simulink model "modelo_real"  (R2018b)
settings: Solver=ode4  StartTime=0.0  StopTime=t_f  FixedStep=fst  RelTol=1e-3  EnableMultiTasking=on
values from neighbouring files (symbols this model uses):
  b = 0.1210    (= 0.121)    [Script_principal.m]
  c_d = r_d/(2*b)    (= 0.120661157025)    [Script_principal.m]
  c_e = r_e/(2*b)    (= 0.121074380165)    [Script_principal.m]
  delayD = 0.1/fst    (= 100)    [Script_principal.m]
  delayE = 0.1/fst    (= 100)    [Script_principal.m]
  fD_v = var_fD*0.0069    (= 0.0069)    [Script_principal.m]
  fE_v = var_fE*0.0053    (= 0.0053)    [Script_principal.m]
  filter_order = 2    [Script_principal.m]
  freq_pos = 200    [Script_principal.m]
  freq_vel = 200    [Script_principal.m]
  I_v = var_I*0.0903    (= 0.0903)    [Script_principal.m]
  Ir_v = var_Ir*0.00094    (= 0.00094)    [Script_principal.m]
  k0 = 25    [Script_principal.m]
  k1 = 25    [Script_principal.m]
  k_enc = 2*pi/fpr    (= 0.157079632679)    [Script_principal.m]
  KaD_v = var_KaD*0.4713    (= 0.4713)    [Script_principal.m]
  KaE_v = var_KaE*0.5046    (= 0.5046)    [Script_principal.m]
  KtD_v = var_KtD*KaD    (= 0.4713)    [Script_principal.m]
  KtE_v = var_KtE*KaE    (= 0.5046)    [Script_principal.m]
  L = 0.10    (= 0.1)    [Script_principal.m]
  m_v = var_m*1.932    (= 1.932)    [Script_principal.m]
  r_d = 0.0292    [Script_principal.m]
  r_e = 0.0293    [Script_principal.m]
  RaD_v = var_RaD*8.4507    (= 8.4507)    [Script_principal.m]
  RaE_v = var_RaE*7.7177    (= 7.7177)    [Script_principal.m]
  svzD = 0    [Script_principal.m]
  svzE = 0    [Script_principal.m]
  T = 4    [Script_principal.m]
  VaD_max = 14    [Script_principal.m]
  VaD_min = 2    [Script_principal.m]
  VaE_max = 14    [Script_principal.m]
  VaE_min = 2    [Script_principal.m]
  x0_1 = 0    [Script_principal.m]
  x0_2 = -L    (= -0.1)    [Script_principal.m]
  x0_3 = (pi/2)/c_d    (= 13.0182435303)    [Script_principal.m]
  x0_4 = 0    [Script_principal.m]
  x0_5 = 0    [Script_principal.m]
  x0_6 = 0    [Script_principal.m]
undefined symbols (not defined in the file or in its folder): a, dur_c, t_f, t_i, t_i_1, t_i_2, t_i_3, t_i_c, time_c, v, w, wx, wy
libraries: simulink x39, embdlinuxlib x7, dspmtrx3 x6, cstblocks x4, raspberrypilib x1
(part 1 of 2)
settings Model: SimulationMode=external  ExtModeTrigDuration=2  Creator=nenem  LastModifiedBy=nenem
settings SolverCC: PositivePriorityOrder=on
settings OptimizationCC: EnhancedBackFolding=on  PassReuseOutputArgsAs=Individual arguments  MaxStackSize=64  OptimizeBlockOrder=speed  DifferentSizesBufferReuse=on  OptimizationCustomize=off
settings DebuggingCC: ParameterTunabilityLossMsg=error
settings HardwareCC: ProdBitPerPointer=32  ProdBitPerSizeT=32  ProdBitPerPtrDiffT=32  ProdLargestAtomicInteger=Long  ProdLargestAtomicFloat=Double  ProdWordSize=32  ProdHWDeviceType=ARM Compatible->ARM Cortex
settings SFSimCC: MATLABDynamicMemAlloc=off
settings RTWCC: SystemTargetFile=ert.tlc  HardwareBoard=Raspberry Pi  TLCOptions="-aInlineSetEventsForThisBaseRateFcn=TLC_FALSE -aSuppressMultiTaskScheduler=TLC_FALSE  -aRateBasedStepFcn=0"  TemplateMakefile=ert_default_tmf  GenerateReport=on  Toolchain=GNU GCC Raspberry Pi  BuildConfiguration=Faster Runs  IncludeHyperlinkInReport=on  LaunchReport=on  GenerateTraceInfo=on  GenerateTraceReport=on  GenerateTraceReportSl=on  GenerateTraceReportSf=on  GenerateTraceReportEml=on
settings CodeAppCC: ForceParamTrailComments=on  IgnoreCustomStorageClasses=off  OperatorAnnotations=on  SimulinkDataObjDesc=on  SFDataObjDesc=on  InsertBlockDesc=on
settings ERTTargetCC: SupportContinuousTime=on  SupportVariableSizeSignals=on

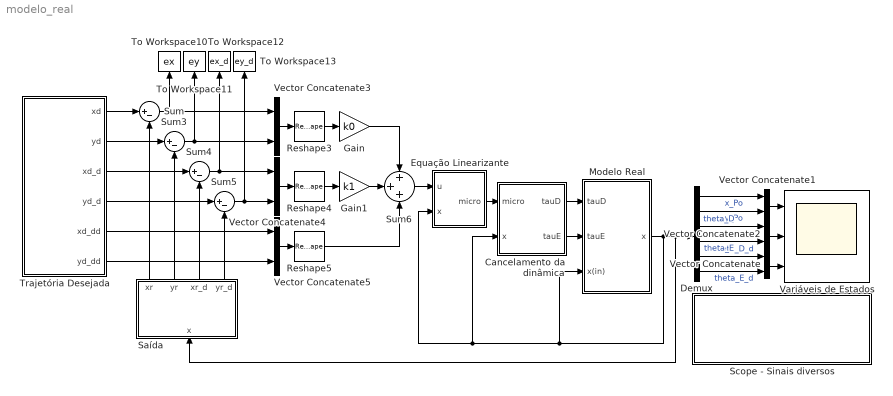
== system modelo_real ==
  Cancelamento da dinâmica : Subsystem
  Demux : Demux  Outputs=6
  Equação Linearizante : Subsystem
  Gain : Gain  Gain=k0
  Gain1 : Gain  Gain=k1
  Modelo Real : Subsystem
  Reshape3 : Reshape  OutputDimensionality=Customize  OutputDimensions=[2,1]
  Reshape4 : Reshape  OutputDimensionality=Customize  OutputDimensions=[2,1]
  Reshape5 : Reshape  OutputDimensionality=Customize  OutputDimensions=[2,1]
  Saída : Subsystem
  Scope - Sinais diversos : Subsystem
  Sum{,3..5} (4 alike) : Sum  Inputs=|+-
  Sum6 : Sum  Inputs=+++
  To Workspace10 : ToWorkspace  VariableName=ex  SaveFormat=Structure With Time  SampleTime=-1
      settings: Save2DSignal=2-D array (concatenate along first dimension)
  To Workspace11 : ToWorkspace  VariableName=ey  SaveFormat=Structure With Time  SampleTime=-1
      settings: Save2DSignal=2-D array (concatenate along first dimension)
  To Workspace12 : ToWorkspace  VariableName=ex_d  SaveFormat=Structure With Time  SampleTime=-1
      settings: Save2DSignal=2-D array (concatenate along first dimension)
  To Workspace13 : ToWorkspace  VariableName=ey_d  SaveFormat=Structure With Time  SampleTime=-1
      settings: Save2DSignal=2-D array (concatenate along first dimension)
  Trajetória Desejada : Subsystem
  Variáveis de Estados : Scope  NumInputPorts=3
  Vector Concatenate{,1..5} (6 alike) : Concatenate
  wires:
  Trajetória Desejada/4(yd_d) -> Sum5/1
  Vector Concatenate5/1 -> Reshape5/1
  Vector Concatenate3/1 -> Reshape3/1
  Vector Concatenate4/1 -> Reshape4/1
  Reshape3/1 -> Gain/1
  Gain/1 -> Sum6/1
  Gain1/1 -> Sum6/2
  Trajetória Desejada/3(xd_d) -> Sum4/1
  Trajetória Desejada/6(yd_dd) -> Vector Concatenate5/2
  Trajetória Desejada/5(xd_dd) -> Vector Concatenate5/1
  Reshape5/1 -> Sum6/3
  Reshape4/1 -> Gain1/1
  Equação Linearizante/1(micro) -> Cancelamento da dinâmica/1(micro)
  Sum6/1 -> Equação Linearizante/1(u)
  Trajetória Desejada/1(xd) -> Sum/1
  Trajetória Desejada/2(yd) -> Sum3/1
  Modelo Real/1(x) -> Saída/1(x), Demux/1, Modelo Real/3(x(in)), Cancelamento da dinâmica/2(x), Equação Linearizante/2(x)
  Vector Concatenate2/1 -> Variáveis de Estados/2
  Vector Concatenate1/1 -> Variáveis de Estados/1
  Vector Concatenate/1 -> Variáveis de Estados/3
  Demux/1 -> Vector Concatenate1/1  "x_Po"
  Demux/2 -> Vector Concatenate1/2  "y_Po"
  Demux/5 -> Vector Concatenate/1  "theta_D_d"
  Demux/6 -> Vector Concatenate/2  "theta_E_d"
  Demux/4 -> Vector Concatenate2/2  "theta_E"
  Demux/3 -> Vector Concatenate2/1  "theta_D"
  Cancelamento da dinâmica/1(tauD) -> Modelo Real/1(tauD)
  Cancelamento da dinâmica/2(tauE) -> Modelo Real/2(tauE)
  Saída/1(xr) -> Sum/2
  Saída/2(yr) -> Sum3/2
  Saída/3(xr_d) -> Sum4/2
  Saída/4(yr_d) -> Sum5/2
  Sum3/1 -> Vector Concatenate3/2, To Workspace11/1
  Sum/1 -> Vector Concatenate3/1, To Workspace10/1
  Sum4/1 -> To Workspace12/1, Vector Concatenate4/1
  Sum5/1 -> Vector Concatenate4/2, To Workspace13/1

== system modelo_real/Cancelamento da dinâmica ==
  micro : Inport
  x : Inport  Port=2
  Constant1 : Constant  Value=[b r_d r_e c_d c_e Ir_v m_v I_v]
  Reshape7 : Reshape  OutputDimensionality=Customize  OutputDimensions=[1,8]
  To Workspace18 : ToWorkspace  VariableName=tauD  SaveFormat=Structure With Time  SampleTime=-1
      settings: Save2DSignal=2-D array (concatenate along first dimension)
  To Workspace19 : ToWorkspace  VariableName=tauE  SaveFormat=Structure With Time  SampleTime=-1
      settings: Save2DSignal=2-D array (concatenate along first dimension)
  Transformação da Entrada : MATLAB Function  TreatAsAtomicUnit=on
  tauD : Outport
  tauE : Outport  Port=2
  tag scope: tauD=global, tauE=global
  wires:
  micro/1 -> Transformação da Entrada/2(micro)
  Constant1/1 -> Reshape7/1
  Reshape7/1 -> Transformação da Entrada/1(cte)
  x/1 -> Transformação da Entrada/3(x)
  Transformação da Entrada/2(tauE) -> tauE/1, To Workspace19/1, [tauE]
  Transformação da Entrada/1(tauD) -> tauD/1, To Workspace18/1, [tauD]

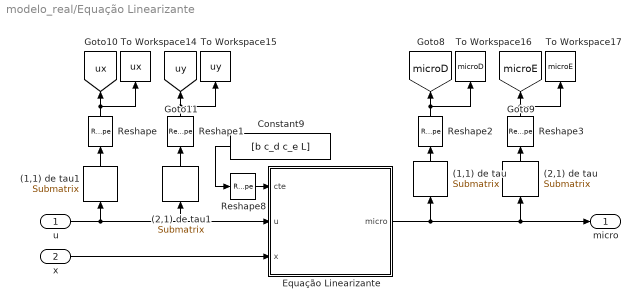
== system modelo_real/Equação Linearizante ==
  u : Inport
  x : Inport  Port=2
  (1,1) de tau : dspmtrx3/Submatrix  RowSpan=One row  RowStartMode=Index  RowStartIndex=1  RowEndMode=Last  RowEndIndex=1  ColSpan=One column  ColStartMode=Index  ColStartIndex=1  ColEndMode=Last  ColEndIndex=1
  (1,1) de tau1 : dspmtrx3/Submatrix  RowSpan=One row  RowStartMode=Index  RowStartIndex=1  RowEndMode=Last  RowEndIndex=1  ColSpan=One column  ColStartMode=Index  ColStartIndex=1  ColEndMode=Last  ColEndIndex=1
  (2,1) de tau : dspmtrx3/Submatrix  RowSpan=One row  RowStartMode=Index  RowStartIndex=2  RowEndMode=Last  RowEndIndex=1  ColSpan=One column  ColStartMode=Index  ColStartIndex=1  ColEndMode=Last  ColEndIndex=1
  (2,1) de tau1 : dspmtrx3/Submatrix  RowSpan=One row  RowStartMode=Index  RowStartIndex=2  RowEndMode=Last  RowEndIndex=1  ColSpan=One column  ColStartMode=Index  ColStartIndex=1  ColEndMode=Last  ColEndIndex=1
  Constant9 : Constant  Value=[b c_d c_e L]
  Equação Linearizante : MATLAB Function  TreatAsAtomicUnit=on
  Reshape{,1..3} (4 alike) : Reshape
  Reshape8 : Reshape  OutputDimensionality=Customize  OutputDimensions=[1,4]
  To Workspace14 : ToWorkspace  VariableName=ux  SaveFormat=Structure With Time  SampleTime=-1
      settings: Save2DSignal=2-D array (concatenate along first dimension)
  To Workspace15 : ToWorkspace  VariableName=uy  SaveFormat=Structure With Time  SampleTime=-1
      settings: Save2DSignal=2-D array (concatenate along first dimension)
  To Workspace16 : ToWorkspace  VariableName=microD  SaveFormat=Structure With Time  SampleTime=-1
      settings: Save2DSignal=2-D array (concatenate along first dimension)
  To Workspace17 : ToWorkspace  VariableName=microE  SaveFormat=Structure With Time  SampleTime=-1
      settings: Save2DSignal=2-D array (concatenate along first dimension)
  micro : Outport
  tag scope: microD=global, microE=global, ux=global, uy=global
  wires:
  Constant9/1 -> Reshape8/1
  Reshape8/1 -> Equação Linearizante/1(cte)
  x/1 -> Equação Linearizante/3(x)
  (2,1) de tau1/1 -> Reshape1/1
  (1,1) de tau1/1 -> Reshape/1
  u/1 -> (1,1) de tau1/1, (2,1) de tau1/1, Equação Linearizante/2(u)
  Reshape/1 -> To Workspace14/1, [ux]
  Reshape1/1 -> To Workspace15/1, [uy]
  Reshape3/1 -> To Workspace17/1, [microE]
  Reshape2/1 -> To Workspace16/1, [microD]
  (2,1) de tau/1 -> Reshape3/1
  Equação Linearizante/1(micro) -> micro/1, (2,1) de tau/1, (1,1) de tau/1
  (1,1) de tau/1 -> Reshape2/1

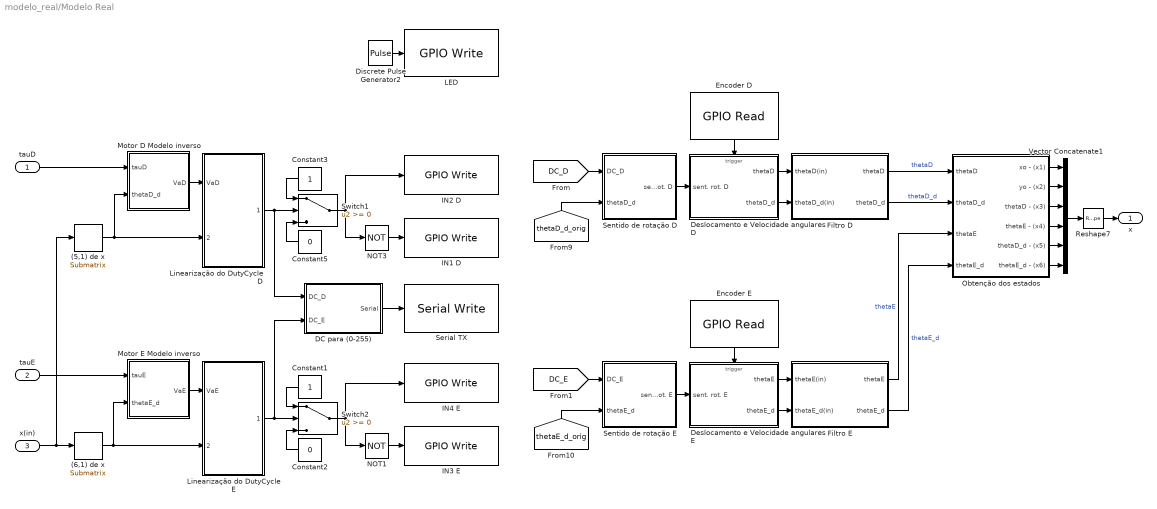
== system modelo_real/Modelo Real ==
  tauD : Inport
  tauE : Inport  Port=2
  x(in) : Inport  Port=3
  (5,1) de x : dspmtrx3/Submatrix  RowSpan=One row  RowStartMode=Index  RowStartIndex=5  RowEndMode=Last  RowEndIndex=1  ColSpan=One column  ColStartMode=Index  ColStartIndex=1  ColEndMode=Last  ColEndIndex=1
  (6,1) de x : dspmtrx3/Submatrix  RowSpan=One row  RowStartMode=Index  RowStartIndex=6  RowEndMode=Last  RowEndIndex=1  ColSpan=One column  ColStartMode=Index  ColStartIndex=1  ColEndMode=Last  ColEndIndex=1
  Constant1 : Constant
  Constant2 : Constant  Value=0
  Constant3 : Constant
  Constant5 : Constant  Value=0
  DC para (0-255) : Subsystem
  Deslocamento e Velocidade angulares D : Subsystem  TreatAsAtomicUnit=on
  Deslocamento e Velocidade angulares E : Subsystem  TreatAsAtomicUnit=on
  Discrete Pulse Generator2 : DiscretePulseGenerator  SampleTime=0.25
  Encoder D : embdlinuxlib/GPIO Read  board=Pi 3 Model B  gpio=26  internalResistor=Off  sampleTime=fst  direction=Input  blockPlatform=Raspberry Pi
      settings: SourceProductName=Simulink Support Package for Raspberry Pi Hardware  SourceProductBaseCode=RASPPI
  Encoder E : embdlinuxlib/GPIO Read  board=Pi 3 Model B  gpio=5  internalResistor=Off  sampleTime=fst  direction=Input  blockPlatform=Raspberry Pi
      settings: SourceProductName=Simulink Support Package for Raspberry Pi Hardware  SourceProductBaseCode=RASPPI
  Filtro D : Subsystem
  Filtro E : Subsystem
  IN1 D : embdlinuxlib/GPIO Write  board=Pi 3 Model B  gpio=16  direction=Output  blockPlatform=Raspberry Pi
      settings: SourceProductName=Simulink Support Package for Raspberry Pi Hardware  SourceProductBaseCode=RASPPI
  IN2 D : embdlinuxlib/GPIO Write  board=Pi 3 Model B  gpio=20  direction=Output  blockPlatform=Raspberry Pi
      settings: SourceProductName=Simulink Support Package for Raspberry Pi Hardware  SourceProductBaseCode=RASPPI
  IN3 E : embdlinuxlib/GPIO Write  board=Pi 3 Model B  gpio=19  direction=Output  blockPlatform=Raspberry Pi
      settings: SourceProductName=Simulink Support Package for Raspberry Pi Hardware  SourceProductBaseCode=RASPPI
  IN4 E : embdlinuxlib/GPIO Write  board=Pi 3 Model B  gpio=6  direction=Output  blockPlatform=Raspberry Pi
      settings: SourceProductName=Simulink Support Package for Raspberry Pi Hardware  SourceProductBaseCode=RASPPI
  LED : embdlinuxlib/GPIO Write  board=Pi 3 Model B  gpio=21  direction=Output  blockPlatform=Raspberry Pi
      settings: SourceProductName=Simulink Support Package for Raspberry Pi Hardware  SourceProductBaseCode=RASPPI
  Linearização do DutyCycle D : Subsystem
  Linearização do DutyCycle E : Subsystem
  Motor D Modelo inverso : Subsystem
  Motor E Modelo inverso : Subsystem
  NOT1 : Logic  Operator=NOT  IconShape=distinctive  AllPortsSameDT=off  OutDataTypeStr=boolean
  NOT3 : Logic  Operator=NOT  IconShape=distinctive  AllPortsSameDT=off  OutDataTypeStr=boolean
  Obtenção dos estados : Subsystem
  Reshape7 : Reshape  OutputDimensionality=Customize  OutputDimensions=[6,1]
  Sentido de rotação D : Subsystem
  Sentido de rotação E : Subsystem
  Serial TX : raspberrypilib/Serial Write  board=Pi 3 Model B  SCIModule_=/dev/ttyS0  Baudrate_=230400  Parity=None  StopBits_=1  HardwareFlowControl=None  ByteOrder=LittleEndian  OutputStatus=off  blockPlatform=RaspberryPi
      settings: SourceProductName=Simulink Support Package for Raspberry Pi Hardware  SourceProductBaseCode=RASPPI
  Switch1 : Switch
  Switch2 : Switch
  Vector Concatenate1 : Concatenate  NumInputs=6
  x : Outport
  wires:
  Filtro D/1(thetaD) -> Obtenção dos estados/1(thetaD)  "thetaD"
  Filtro E/1(thetaE) -> Obtenção dos estados/3(thetaE)  "thetaE"
  Sentido de rotação D/1(sent. rot. D) -> Deslocamento e Velocidade angulares D/1(sent. rot. D)
  Sentido de rotação E/1(sent. rot. E) -> Deslocamento e Velocidade angulares E/1(sent. rot. E)
  Encoder E/1 -> Deslocamento e Velocidade angulares E/Trigger
  [DC_D] -> Sentido de rotação D/1(DC_D)
  Encoder D/1 -> Deslocamento e Velocidade angulares D/Trigger
  Discrete Pulse Generator2/1 -> LED/1
  Vector Concatenate1/1 -> Reshape7/1
  Filtro D/2(thetaD_d) -> Obtenção dos estados/2(thetaD_d)  "thetaD_d"
  Filtro E/2(thetaE_d) -> Obtenção dos estados/4(thetaE_d)  "thetaE_d"
  [DC_E] -> Sentido de rotação E/1(DC_E)
  tauD/1 -> Motor D Modelo inverso/1(tauD)
  (5,1) de x/1 -> Motor D Modelo inverso/2(thetaD_d), Linearização do DutyCycle D/2(thetaD_d)
  Motor D Modelo inverso/1(VaD) -> Linearização do DutyCycle D/1(VaD)
  tauE/1 -> Motor E Modelo inverso/1(tauE)
  Motor E Modelo inverso/1(VaE) -> Linearização do DutyCycle E/1(VaE)
  (6,1) de x/1 -> Motor E Modelo inverso/2(thetaE_d), Linearização do DutyCycle E/2(thetaE_d)
  DC para (0-255)/1(Serial) -> Serial TX/1
  Constant3/1 -> Switch1/1
  Constant5/1 -> Switch1/3
  Constant1/1 -> Switch2/1
  Constant2/1 -> Switch2/3
  Deslocamento e Velocidade angulares D/1(thetaD) -> Filtro D/1(thetaD(in))
  Deslocamento e Velocidade angulares D/2(thetaD_d) -> Filtro D/2(thetaD_d(in))
  Deslocamento e Velocidade angulares E/1(thetaE) -> Filtro E/1(thetaE(in))
  Deslocamento e Velocidade angulares E/2(thetaE_d) -> Filtro E/2(thetaE_d(in))
  Reshape7/1 -> x/1
  x(in)/1 -> (5,1) de x/1, (6,1) de x/1
  Obtenção dos estados/1(xo - (x1)) -> Vector Concatenate1/1
  Obtenção dos estados/2(yo - (x2)) -> Vector Concatenate1/2
  Obtenção dos estados/3(thetaD - (x3)) -> Vector Concatenate1/3
  Obtenção dos estados/4(thetaE - (x4)) -> Vector Concatenate1/4
  Obtenção dos estados/5(thetaD_d - (x5)) -> Vector Concatenate1/5
  Obtenção dos estados/6(thetaE_d - (x6)) -> Vector Concatenate1/6
  [thetaE_d_orig] -> Sentido de rotação E/2(thetaE_d)
  [thetaD_d_orig] -> Sentido de rotação D/2(thetaD_d)
  Linearização do DutyCycle D/1(DutyCycleD) -> DC para (0-255)/1(DC_D), Switch1/2
  Linearização do DutyCycle E/1(DutyCycleE) -> DC para (0-255)/2(DC_E), Switch2/2
  Switch1/1 -> IN2 D/1, NOT3/1
  NOT3/1 -> IN1 D/1
  Switch2/1 -> IN4 E/1, NOT1/1
  NOT1/1 -> IN3 E/1

== system modelo_real/Saída ==
  x : Inport
  Constant9 : Constant  Value=[b c_d c_e L]
  Hypot2 : Math  Operator=hypot  SaturateOnIntegerOverflow=on
  Reshape1 : Reshape  OutputDimensionality=Customize  OutputDimensions=[6,1]
  Reshape9 : Reshape  OutputDimensionality=Customize  OutputDimensions=[1,4]
  Saídas : MATLAB Function  TreatAsAtomicUnit=on
  To Workspace3 : ToWorkspace  VariableName=xr  SaveFormat=Structure With Time  SampleTime=-1
      settings: Save2DSignal=2-D array (concatenate along first dimension)
  To Workspace4 : ToWorkspace  VariableName=yr  SaveFormat=Structure With Time  SampleTime=-1
      settings: Save2DSignal=2-D array (concatenate along first dimension)
  To Workspace7 : ToWorkspace  VariableName=vr  SaveFormat=Structure With Time  SampleTime=-1
      settings: Save2DSignal=2-D array (concatenate along first dimension)
  xr : Outport
  yr : Outport  Port=2
  xr_d : Outport  Port=3
  yr_d : Outport  Port=4
  wires:
  Reshape9/1 -> Saídas/1(cte)
  Constant9/1 -> Reshape9/1
  x/1 -> Reshape1/1
  Saídas/3(xr_d) -> xr_d/1, Hypot2/1
  Saídas/4(yr_d) -> yr_d/1, Hypot2/2
  Saídas/1(xr) -> xr/1, To Workspace3/1
  Saídas/2(yr) -> yr/1, To Workspace4/1
  Hypot2/1 -> To Workspace7/1
  Reshape1/1 -> Saídas/2(x)

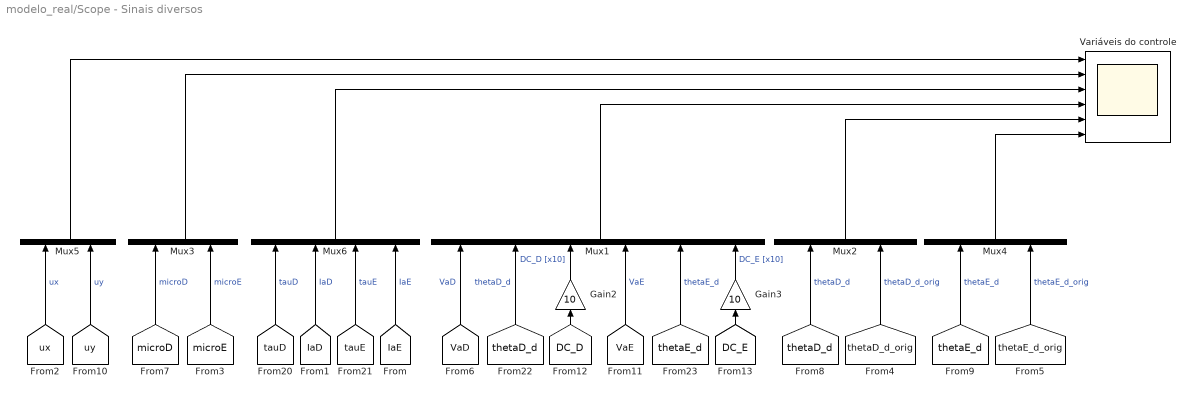
== system modelo_real/Scope - Sinais diversos ==
  Gain2 : Gain  Gain=10
  Gain3 : Gain  Gain=10
  Mux1 : Mux  Inputs=6
  Mux{2..5} (4 alike) : Mux  Inputs=2
  Mux6 : Mux
  Variáveis do controle : Scope  NumInputPorts=6
  wires:
  [microE] -> Mux3/2  "microE"
  Gain3/1 -> Mux1/6  "DC_E [x10]"
  [ux] -> Mux5/1  "ux"
  [uy] -> Mux5/2  "uy"
  Mux2/1 -> Variáveis do controle/5
  [thetaD_d] -> Mux1/2  "thetaD_d"
  [microD] -> Mux3/1  "microD"
  [VaE] -> Mux1/4  "VaE"
  [DC_E] -> Gain3/1
  [DC_D] -> Gain2/1
  [thetaE_d] -> Mux1/5  "thetaE_d"
  Gain2/1 -> Mux1/3  "DC_D [x10]"
  [VaD] -> Mux1/1  "VaD"
  Mux3/1 -> Variáveis do controle/2
  Mux6/1 -> Variáveis do controle/3
  Mux5/1 -> Variáveis do controle/1
  Mux4/1 -> Variáveis do controle/6
  Mux1/1 -> Variáveis do controle/4
  [IaD] -> Mux6/2  "IaD"
  [tauE] -> Mux6/3  "tauE"
  [tauD] -> Mux6/1  "tauD"
  [IaE] -> Mux6/4  "IaE"
  [thetaD_d_orig] -> Mux2/2  "thetaD_d_orig"
  [thetaD_d] -> Mux2/1  "thetaD_d"
  [thetaE_d_orig] -> Mux4/2  "thetaE_d_orig"
  [thetaE_d] -> Mux4/1  "thetaE_d"

== system modelo_real/Trajetória Desejada ==
  Derivative3 : Derivative
  Derivative4 : Derivative
  Hypot : Math  Operator=hypot  OutputSignalType=real  SaturateOnIntegerOverflow=on
  Integrator : Integrator
  Integrator1 : Integrator
  To Workspace : ToWorkspace  VariableName=vd  SaveFormat=Structure With Time  SampleTime=-1
      settings: Save2DSignal=2-D array (concatenate along first dimension)
  To Workspace1 : ToWorkspace  VariableName=xd  SaveFormat=Structure With Time  SampleTime=-1
      settings: Save2DSignal=2-D array (concatenate along first dimension)
  To Workspace2 : ToWorkspace  VariableName=yd  SaveFormat=Structure With Time  SampleTime=-1
      settings: Save2DSignal=2-D array (concatenate along first dimension)
  To Workspace5 : ToWorkspace  VariableName=xd_d  SaveFormat=Structure With Time  SampleTime=-1
      settings: Save2DSignal=2-D array (concatenate along first dimension)
  To Workspace6 : ToWorkspace  VariableName=yd_d  SaveFormat=Structure With Time  SampleTime=-1
      settings: Save2DSignal=2-D array (concatenate along first dimension)
  To Workspace8 : ToWorkspace  VariableName=xd_dd  SaveFormat=Structure With Time  SampleTime=-1
      settings: Save2DSignal=2-D array (concatenate along first dimension)
  To Workspace9 : ToWorkspace  VariableName=yd_dd  SaveFormat=Structure With Time  SampleTime=-1
      settings: Save2DSignal=2-D array (concatenate along first dimension)
  Velocidade da trajetória : Subsystem
  xd : Outport
  yd : Outport  Port=2
  xd_d : Outport  Port=3
  yd_d : Outport  Port=4
  xd_dd : Outport  Port=5
  yd_dd : Outport  Port=6
  wires:
  Derivative3/1 -> xd_dd/1, To Workspace8/1  "xd_dd"
  Derivative4/1 -> yd_dd/1, To Workspace9/1  "yd_dd"
  Integrator/1 -> xd/1, To Workspace1/1  "xd"
  Integrator1/1 -> yd/1, To Workspace2/1  "yd"
  Hypot/1 -> To Workspace/1
  Velocidade da trajetória/1(xd_d) -> Integrator/1, Derivative3/1, xd_d/1, To Workspace5/1, Hypot/1  "xd_d"
  Velocidade da trajetória/2(yd_d) -> Integrator1/1, yd_d/1, To Workspace6/1, Hypot/2, Derivative4/1  "yd_d"

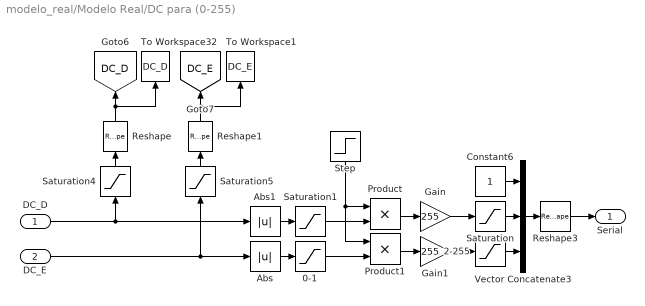
== system modelo_real/Modelo Real/DC para (0-255) ==
  DC_D : Inport
  DC_E : Inport  Port=2
  0-1 : Saturate  UpperLimit=1  LowerLimit=0
  2-255 : Saturate  UpperLimit=255  LowerLimit=2
  Abs : Abs
  Abs1 : Abs
  Constant6 : Constant  OutDataTypeStr=uint8
  Gain : Gain  Gain=255  OutDataTypeStr=uint8
  Gain1 : Gain  Gain=255  OutDataTypeStr=uint8
  Product : Product
  Product1 : Product
  Reshape : Reshape
  Reshape1 : Reshape
  Reshape3 : Reshape  OutputDimensionality=Column vector (2-D)  OutputDimensions=[3,1]
  Saturation : Saturate  UpperLimit=255  LowerLimit=2
  Saturation1 : Saturate  UpperLimit=1  LowerLimit=0
  Saturation4 : Saturate  UpperLimit=1  LowerLimit=-1
  Saturation5 : Saturate  UpperLimit=1  LowerLimit=-1
  Step : Step  Time=t_f-0.01  Before=1  After=0  SampleTime=0
  To Workspace1 : ToWorkspace  VariableName=DC_E  SaveFormat=Structure With Time  SampleTime=-1
      settings: Save2DSignal=2-D array (concatenate along first dimension)
  To Workspace32 : ToWorkspace  VariableName=DC_D  SaveFormat=Structure With Time  SampleTime=-1
      settings: Save2DSignal=2-D array (concatenate along first dimension)
  Vector Concatenate3 : Concatenate  NumInputs=3  ConcatenateDimension=5
  Serial : Outport
  tag scope: DC_D=global, DC_E=global
  wires:
  DC_E/1 -> Abs/1, Saturation5/1
  Saturation/1 -> Vector Concatenate3/2
  DC_D/1 -> Abs1/1, Saturation4/1
  Constant6/1 -> Vector Concatenate3/1
  2-255/1 -> Vector Concatenate3/3
  Vector Concatenate3/1 -> Reshape3/1
  Reshape3/1 -> Serial/1
  Saturation4/1 -> Reshape/1
  Saturation5/1 -> Reshape1/1
  Abs/1 -> 0-1/1
  Abs1/1 -> Saturation1/1
  0-1/1 -> Product1/2
  Saturation1/1 -> Product/2
  Reshape/1 -> To Workspace32/1, [DC_D]
  Reshape1/1 -> To Workspace1/1, [DC_E]
  Gain/1 -> Saturation/1
  Gain1/1 -> 2-255/1
  Step/1 -> Product1/1, Product/1
  Product/1 -> Gain/1
  Product1/1 -> Gain1/1

== system modelo_real/Modelo Real/Deslocamento e Velocidade angulares D ==
  sent. rot. D : Inport  LatchByDelayingOutsideSignal=on
  Trigger : TriggerPort  VariantControl=Variant
  Add2 : Sum  Inputs=|+-
  Constant1 : Constant  OutDataTypeStr=double
  Constant9 : Constant  Value=0  OutDataTypeStr=double
  Digital Clock : DigitalClock  SampleTime=-1
  Fcn : Fcn  Expr=u^(-1)
  Gain : Gain  Gain=k_enc
  Gain1 : Gain  Gain=k_enc
  Product1 : Product
  Product3 : Product
  Sum1 : Sum  Inputs=|++
  Sum2 : Sum  Inputs=+-|
  Switch1 : Switch  Criteria=u2 ~= 0
  Unit Delay1 : UnitDelay  SampleTime=-1
  Unit Delay2 : UnitDelay  SampleTime=-1
  thetaD : Outport
  thetaD_d : Outport  Port=2
  wires:
  Constant1/1 -> Product1/2, Add2/2
  Sum1/1 -> Unit Delay1/1, Add2/1
  Add2/1 -> Gain1/1
  Unit Delay1/1 -> Sum1/2
  Product1/1 -> Sum1/1
  Fcn/1 -> Gain/1
  Digital Clock/1 -> Unit Delay2/1, Sum2/1
  Constant9/1 -> Switch1/3
  Unit Delay2/1 -> Switch1/2, Sum2/2
  Switch1/1 -> Product3/2
  Sum2/1 -> Fcn/1
  sent. rot. D/1 -> Product1/1, Product3/1
  Gain/1 -> Switch1/1
  Product3/1 -> thetaD_d/1
  Gain1/1 -> thetaD/1

== system modelo_real/Modelo Real/Deslocamento e Velocidade angulares E ==
  sent. rot. E : Inport  LatchByDelayingOutsideSignal=on
  Trigger : TriggerPort  VariantControl=Variant
  Add2 : Sum  Inputs=|+-
  Constant1 : Constant  OutDataTypeStr=double
  Constant9 : Constant  Value=0  OutDataTypeStr=double
  Digital Clock : DigitalClock  SampleTime=-1
  Fcn : Fcn  Expr=u^(-1)
  Gain : Gain  Gain=k_enc
  Gain1 : Gain  Gain=k_enc
  Product1 : Product
  Product3 : Product
  Sum1 : Sum  Inputs=|++
  Sum2 : Sum  Inputs=+-|
  Switch1 : Switch  Criteria=u2 ~= 0
  Unit Delay1 : UnitDelay  SampleTime=-1
  Unit Delay2 : UnitDelay  SampleTime=-1
  thetaE : Outport
  thetaE_d : Outport  Port=2
  wires:
  Constant1/1 -> Product1/2, Add2/2
  Sum1/1 -> Unit Delay1/1, Add2/1
  Add2/1 -> Gain1/1
  Unit Delay1/1 -> Sum1/2
  Product1/1 -> Sum1/1
  Fcn/1 -> Gain/1
  Digital Clock/1 -> Unit Delay2/1, Sum2/1
  Constant9/1 -> Switch1/3
  Unit Delay2/1 -> Switch1/2, Sum2/2
  Switch1/1 -> Product3/2
  Sum2/1 -> Fcn/1
  sent. rot. E/1 -> Product1/1, Product3/1
  Gain/1 -> Switch1/1
  Product3/1 -> thetaE_d/1
  Gain1/1 -> thetaE/1

== system modelo_real/Modelo Real/Filtro D ==
  thetaD(in) : Inport
  thetaD_d(in) : Inport  Port=2
  Constant : Constant  Value=freq_vel
  Constant1 : Constant  Value=freq_pos
  Constant6 : Constant  Value=0
  Manual Switch : ManualSwitch  CurrentSetting=0
  Média : MATLAB Function  TreatAsAtomicUnit=on
  Sum : Sum  Inputs=+-|
  Switch3 : Switch  Criteria=u2 ~= 0
  Tapped Delay : simulink/Discrete/Tapped Delay  vinit=0.0  samptime=fst  NumDelays=delayD  DelayOrder=Oldest  includeCurrent=off
  To Workspace1 : ToWorkspace  VariableName=thetaD_orig  SaveFormat=Structure With Time  SampleTime=-1
      settings: Save2DSignal=2-D array (concatenate along first dimension)
  To Workspace32 : ToWorkspace  VariableName=thetaD_d_orig  SaveFormat=Structure With Time  SampleTime=-1
      settings: Save2DSignal=2-D array (concatenate along first dimension)
  Unit Delay2 : UnitDelay  SampleTime=-1
  Varying Lowpass Filter : cstblocks/Linear Parameter Varying/Varying Lowpass Filter  N=filter_order
      settings: SourceProductName=Control System Toolbox
  Varying Lowpass Filter1 : cstblocks/Linear Parameter Varying/Varying Lowpass Filter  N=filter_order
      settings: SourceProductName=Control System Toolbox
  thetaD : Outport
  thetaD_d : Outport  Port=2
  tag scope: thetaD_d_orig=global
  wires:
  Constant6/1 -> Switch3/3
  Média/1(y) -> Sum/1, Unit Delay2/1
  thetaD_d(in)/1 -> Switch3/1
  Tapped Delay/1 -> Média/1(u)
  Unit Delay2/1 -> Sum/2
  Sum/1 -> Switch3/2  "Δpos"
  Constant/1 -> Varying Lowpass Filter/2
  Switch3/1 -> Varying Lowpass Filter/1, [thetaD_d_orig], To Workspace32/1
  Varying Lowpass Filter/1 -> thetaD_d/1
  Constant1/1 -> Varying Lowpass Filter1/2
  thetaD(in)/1 -> Manual Switch/1, Varying Lowpass Filter1/1, To Workspace1/1, Tapped Delay/1
  Manual Switch/1 -> thetaD/1
  Varying Lowpass Filter1/1 -> Manual Switch/2

== system modelo_real/Modelo Real/Filtro E ==
  thetaE(in) : Inport
  thetaE_d(in) : Inport  Port=2
  Constant : Constant  Value=freq_vel
  Constant1 : Constant  Value=freq_pos
  Constant6 : Constant  Value=0
  Manual Switch : ManualSwitch  CurrentSetting=0
  Média : MATLAB Function  TreatAsAtomicUnit=on
  Sum : Sum  Inputs=+-|
  Switch3 : Switch  Criteria=u2 ~= 0
  Tapped Delay : simulink/Discrete/Tapped Delay  vinit=0.0  samptime=fst  NumDelays=delayE  DelayOrder=Oldest  includeCurrent=off
  To Workspace1 : ToWorkspace  VariableName=thetaE_orig  SaveFormat=Structure With Time  SampleTime=-1
      settings: Save2DSignal=2-D array (concatenate along first dimension)
  To Workspace33 : ToWorkspace  VariableName=thetaE_d_orig  SaveFormat=Structure With Time  SampleTime=-1
      settings: Save2DSignal=2-D array (concatenate along first dimension)
  Unit Delay2 : UnitDelay  SampleTime=-1
  Varying Lowpass Filter : cstblocks/Linear Parameter Varying/Varying Lowpass Filter  N=filter_order
      settings: SourceProductName=Control System Toolbox
  Varying Lowpass Filter1 : cstblocks/Linear Parameter Varying/Varying Lowpass Filter  N=filter_order
      settings: SourceProductName=Control System Toolbox
  thetaE : Outport
  thetaE_d : Outport  Port=2
  tag scope: thetaE_d_orig=global
  wires:
  Constant6/1 -> Switch3/3
  Média/1(y) -> Sum/1, Unit Delay2/1
  thetaE_d(in)/1 -> Switch3/1
  Tapped Delay/1 -> Média/1(u)
  Unit Delay2/1 -> Sum/2
  Sum/1 -> Switch3/2  "Δpos"
  Constant/1 -> Varying Lowpass Filter/2
  Switch3/1 -> Varying Lowpass Filter/1, [thetaE_d_orig], To Workspace33/1
  Varying Lowpass Filter/1 -> thetaE_d/1
  Constant1/1 -> Varying Lowpass Filter1/2
  thetaE(in)/1 -> To Workspace1/1, Manual Switch/1, Varying Lowpass Filter1/1, Tapped Delay/1
  Manual Switch/1 -> thetaE/1
  Varying Lowpass Filter1/1 -> Manual Switch/2

== system modelo_real/Modelo Real/Linearização do DutyCycle D ==
  VaD : Inport
  thetaD_d : Inport  Port=2
  Abs : Abs
  Constant : Constant  Value=VaD_max
  Constant1 : Constant  Value=VaD_max
  Constant3 : Constant
  Constant5 : Constant  Value=-1
  Divide1 : Product  Inputs=*/
  Gain1 : Gain  Gain=KaD_v
  Manual Switch : ManualSwitch  CurrentSetting=0
  Product : Product
  Product1 : Product  Inputs=/*
  Sum1 : Sum  Inputs=|+-
  Sum2 : Sum  Inputs=|+-
  Switch1 : Switch
  DutyCycleD : Outport
  wires:
  Sum2/1 -> Abs/1
  Constant5/1 -> Switch1/3
  Product/1 -> Sum2/1
  Sum1/1 -> Divide1/1
  thetaD_d/1 -> Gain1/1
  Constant/1 -> Product/1
  VaD/1 -> Switch1/2, Product1/2, Sum1/1
  Switch1/1 -> Product/2
  Constant3/1 -> Switch1/1
  Gain1/1 -> Sum1/2, Sum2/2  "f.c.e.m."
  Abs/1 -> Divide1/2
  Divide1/1 -> Manual Switch/2
  Constant1/1 -> Product1/1
  Product1/1 -> Manual Switch/1
  Manual Switch/1 -> DutyCycleD/1

== system modelo_real/Modelo Real/Linearização do DutyCycle E ==
  VaE : Inport
  thetaE_d : Inport  Port=2
  Abs : Abs
  Constant1 : Constant  Value=-1
  Constant2 : Constant  Value=VaD_max
  Constant3 : Constant
  Constant5 : Constant  Value=VaE_max
  Divide : Product  Inputs=*/
  Gain12 : Gain  Gain=KaE_v
  Manual Switch : ManualSwitch  CurrentSetting=0
  Product : Product
  Product1 : Product  Inputs=/*
  Sum4 : Sum  Inputs=|+-
  Sum5 : Sum  Inputs=|+-
  Switch1 : Switch
  DutyCycleE : Outport
  wires:
  thetaE_d/1 -> Gain12/1
  Constant3/1 -> Switch1/1
  Constant5/1 -> Product/1
  Product/1 -> Sum5/1
  Constant1/1 -> Switch1/3
  Sum4/1 -> Divide/1
  Gain12/1 -> Sum4/2, Sum5/2  "f.c.e.m."
  Abs/1 -> Divide/2
  Sum5/1 -> Abs/1
  Switch1/1 -> Product/2
  Constant2/1 -> Product1/1
  VaE/1 -> Sum4/1, Product1/2, Switch1/2
  Product1/1 -> Manual Switch/1
  Divide/1 -> Manual Switch/2
  Manual Switch/1 -> DutyCycleE/1

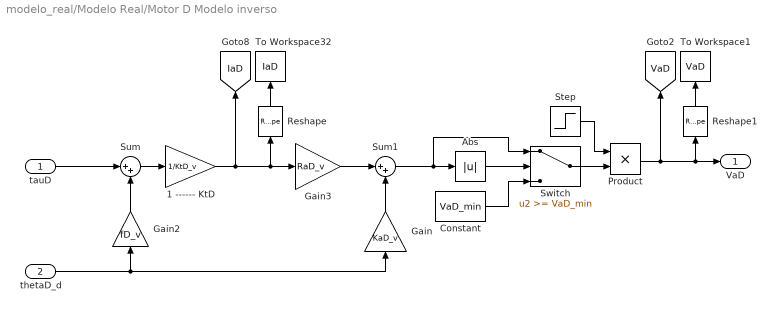
== system modelo_real/Modelo Real/Motor D Modelo inverso ==
  tauD : Inport
  thetaD_d : Inport  Port=2
  1 ------ KtD : Gain  Gain=1/KtD_v
  Abs : Abs
  Constant : Constant  Value=VaD_min
  Gain : Gain  Gain=KaD_v
  Gain2 : Gain  Gain=fD_v
  Gain3 : Gain  Gain=RaD_v
  Product : Product
  Reshape : Reshape
  Reshape1 : Reshape
  Step : Step  Time=t_i  SampleTime=0
  Sum : Sum  Inputs=|++
  Sum1 : Sum  Inputs=|++
  Switch : Switch  Threshold=VaD_min
  To Workspace1 : ToWorkspace  VariableName=VaD  SaveFormat=Structure With Time  SampleTime=-1
      settings: Save2DSignal=2-D array (concatenate along first dimension)
  To Workspace32 : ToWorkspace  VariableName=IaD  SaveFormat=Structure With Time  SampleTime=-1
      settings: Save2DSignal=2-D array (concatenate along first dimension)
  VaD : Outport
  tag scope: IaD=global, VaD=global
  wires:
  Gain2/1 -> Sum/2
  tauD/1 -> Sum/1
  Sum1/1 -> Switch/1, Abs/1
  1 ------ KtD/1 -> Reshape/1, Gain3/1, [IaD]
  Sum/1 -> 1 ------ KtD/1
  Gain3/1 -> Sum1/1
  thetaD_d/1 -> Gain2/1, Gain/1
  Gain/1 -> Sum1/2
  Reshape/1 -> To Workspace32/1
  Reshape1/1 -> To Workspace1/1
  Product/1 -> [VaD], VaD/1, Reshape1/1
  Abs/1 -> Switch/2
  Constant/1 -> Switch/3
  Step/1 -> Product/1
  Switch/1 -> Product/2

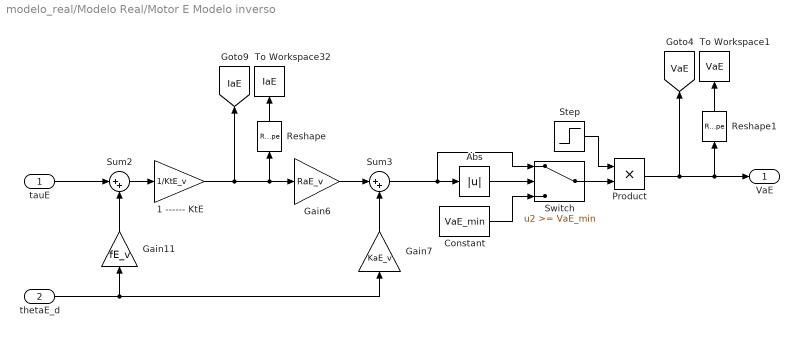
== system modelo_real/Modelo Real/Motor E Modelo inverso ==
  tauE : Inport
  thetaE_d : Inport  Port=2
  1 ------ KtE : Gain  Gain=1/KtE_v
  Abs : Abs
  Constant : Constant  Value=VaE_min
  Gain11 : Gain  Gain=fE_v
  Gain6 : Gain  Gain=RaE_v
  Gain7 : Gain  Gain=KaE_v
  Product : Product
  Reshape : Reshape
  Reshape1 : Reshape
  Step : Step  Time=t_i  SampleTime=0
  Sum2 : Sum  Inputs=|++
  Sum3 : Sum  Inputs=|++
  Switch : Switch  Threshold=VaE_min
  To Workspace1 : ToWorkspace  VariableName=VaE  SaveFormat=Structure With Time  SampleTime=-1
      settings: Save2DSignal=2-D array (concatenate along first dimension)
  To Workspace32 : ToWorkspace  VariableName=IaE  SaveFormat=Structure With Time  SampleTime=-1
      settings: Save2DSignal=2-D array (concatenate along first dimension)
  VaE : Outport
  tag scope: IaE=global, VaE=global
  wires:
  thetaE_d/1 -> Gain7/1, Gain11/1
  1 ------ KtE/1 -> Reshape/1, Gain6/1, [IaE]
  Gain11/1 -> Sum2/2
  Gain7/1 -> Sum3/2
  tauE/1 -> Sum2/1
  Sum2/1 -> 1 ------ KtE/1
  Gain6/1 -> Sum3/1
  Reshape/1 -> To Workspace32/1
  Reshape1/1 -> To Workspace1/1
  Product/1 -> [VaE], Reshape1/1, VaE/1
  Sum3/1 -> Switch/1, Abs/1
  Abs/1 -> Switch/2
  Constant/1 -> Switch/3
  Step/1 -> Product/1
  Switch/1 -> Product/2

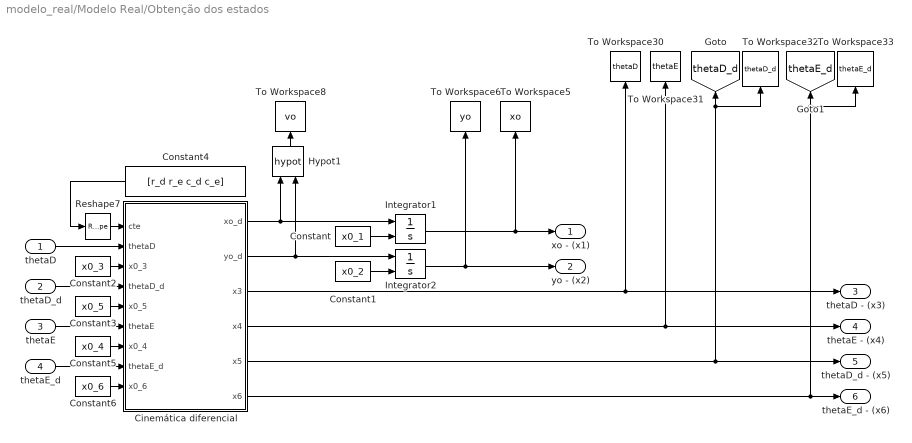
== system modelo_real/Modelo Real/Obtenção dos estados ==
  thetaD : Inport
  thetaD_d : Inport  Port=2
  thetaE : Inport  Port=3
  thetaE_d : Inport  Port=4
  Cinemática diferencial : MATLAB Function  TreatAsAtomicUnit=on
  Constant : Constant  Value=x0_1
  Constant1 : Constant  Value=x0_2
  Constant2 : Constant  Value=x0_3
  Constant3 : Constant  Value=x0_5
  Constant4 : Constant  Value=[r_d r_e c_d c_e]
  Constant5 : Constant  Value=x0_4
  Constant6 : Constant  Value=x0_6
  Hypot1 : Math  Operator=hypot  SaturateOnIntegerOverflow=on
  Integrator1 : Integrator  InitialConditionSource=external  InitialCondition=-0.2
  Integrator2 : Integrator  InitialConditionSource=external  InitialCondition=-0.25
  Reshape7 : Reshape  OutputDimensionality=Customize  OutputDimensions=[1,4]
  To Workspace30 : ToWorkspace  VariableName=thetaD  SaveFormat=Structure With Time  SampleTime=-1
      settings: Save2DSignal=2-D array (concatenate along first dimension)
  To Workspace31 : ToWorkspace  VariableName=thetaE  SaveFormat=Structure With Time  SampleTime=-1
      settings: Save2DSignal=2-D array (concatenate along first dimension)
  To Workspace32 : ToWorkspace  VariableName=thetaD_d  SaveFormat=Structure With Time  SampleTime=-1
      settings: Save2DSignal=2-D array (concatenate along first dimension)
  To Workspace33 : ToWorkspace  VariableName=thetaE_d  SaveFormat=Structure With Time  SampleTime=-1
      settings: Save2DSignal=2-D array (concatenate along first dimension)
  To Workspace5 : ToWorkspace  VariableName=xo  SaveFormat=Structure With Time  SampleTime=-1
      settings: Save2DSignal=2-D array (concatenate along first dimension)
  To Workspace6 : ToWorkspace  VariableName=yo  SaveFormat=Structure With Time  SampleTime=-1
      settings: Save2DSignal=2-D array (concatenate along first dimension)
  To Workspace8 : ToWorkspace  VariableName=vo  SaveFormat=Structure With Time  SampleTime=-1
      settings: Save2DSignal=2-D array (concatenate along first dimension)
  xo - (x1) : Outport
  yo - (x2) : Outport  Port=2
  thetaD - (x3) : Outport  Port=3
  thetaE - (x4) : Outport  Port=4
  thetaD_d - (x5) : Outport  Port=5
  thetaE_d - (x6) : Outport  Port=6
  tag scope: thetaD_d=global, thetaE_d=global
  wires:
  Constant4/1 -> Reshape7/1
  Reshape7/1 -> Cinemática diferencial/1(cte)
  Cinemática diferencial/1(xo_d) -> Hypot1/1, Integrator1/1
  Integrator2/1 -> yo - (x2)/1, To Workspace6/1
  Integrator1/1 -> To Workspace5/1, xo - (x1)/1
  thetaE/1 -> Cinemática diferencial/6(thetaE)
  thetaE_d/1 -> Cinemática diferencial/8(thetaE_d)
  thetaD_d/1 -> Cinemática diferencial/4(thetaD_d)
  thetaD/1 -> Cinemática diferencial/2(thetaD)
  Hypot1/1 -> To Workspace8/1
  Cinemática diferencial/2(yo_d) -> Hypot1/2, Integrator2/1
  Constant/1 -> Integrator1/2
  Constant1/1 -> Integrator2/2
  Constant2/1 -> Cinemática diferencial/3(x0_3)
  Constant6/1 -> Cinemática diferencial/9(x0_6)
  Constant3/1 -> Cinemática diferencial/5(x0_5)
  Constant5/1 -> Cinemática diferencial/7(x0_4)
  Cinemática diferencial/3(x3) -> thetaD - (x3)/1, To Workspace30/1
  Cinemática diferencial/4(x4) -> thetaE - (x4)/1, To Workspace31/1
  Cinemática diferencial/5(x5) -> thetaD_d - (x5)/1, To Workspace32/1, [thetaD_d]
  Cinemática diferencial/6(x6) -> To Workspace33/1, [thetaE_d], thetaE_d - (x6)/1

== system modelo_real/Modelo Real/Sentido de rotação D ==
  DC_D : Inport
  thetaD_d : Inport  Port=2
  Abs : Abs
  Constant1 : Constant  Value=-1  OutDataTypeStr=double
  Constant4 : Constant  OutDataTypeStr=double
  Switch : Switch  Criteria=u2 > Threshold  Threshold=svzD
  Switch1 : Switch
  sent. rot. D : Outport
  wires:
  thetaD_d/1 -> Switch/1, Abs/1
  Switch1/1 -> sent. rot. D/1
  Switch/1 -> Switch1/2
  DC_D/1 -> Switch/3
  Constant4/1 -> Switch1/1
  Constant1/1 -> Switch1/3
  Abs/1 -> Switch/2

== system modelo_real/Modelo Real/Sentido de rotação E ==
  DC_E : Inport
  thetaE_d : Inport  Port=2
  Abs : Abs
  Constant1 : Constant  Value=-1  OutDataTypeStr=double
  Constant4 : Constant  OutDataTypeStr=double
  Switch : Switch  Criteria=u2 > Threshold  Threshold=svzE
  Switch1 : Switch
  sent. rot. E : Outport
  wires:
  Switch1/1 -> sent. rot. E/1
  Switch/1 -> Switch1/2
  DC_E/1 -> Switch/3
  Constant4/1 -> Switch1/1
  Constant1/1 -> Switch1/3
  thetaE_d/1 -> Abs/1, Switch/1
  Abs/1 -> Switch/2

== system modelo_real/Trajetória Desejada/Velocidade da trajetória ==
  Circulo : Subsystem  Commented=on
  Circulo RAMPA : Subsystem  Commented=on
  Constant : Constant  Value=T
  Linha Reta RAMPA : Subsystem  Commented=on
  Multiport Switch : MultiPortSwitch  Inputs=4
  Multiport Switch1 : MultiPortSwitch  Inputs=4
  "Trajetóra em \"L\" Curva 180° suave RAMPA" : Subsystem  Commented=on
  "Trajetóra em \"L\" Curva 90° suave " : Subsystem  Commented=on
  "Trajetóra em \"L\" Curva 90° suave RAMPA" : Subsystem  Commented=on
  Trajetóra em 8 : Subsystem
  xd_d : Outport
  yd_d : Outport  Port=2
  wires:
  Circulo RAMPA/2(yd_d) -> Multiport Switch1/2  "yd_d"
  "Trajetóra em \"L\" Curva 90° suave RAMPA"/2(yd_d) -> Multiport Switch1/3  "yd_d"
  "Trajetóra em \"L\" Curva 90° suave RAMPA"/1(xd_d) -> Multiport Switch/3  "xd_d"
  Circulo RAMPA/1(xd_d) -> Multiport Switch/2  "xd_d"
  Constant/1 -> Multiport Switch/1, Multiport Switch1/1
  Multiport Switch/1 -> xd_d/1  "xd_d"
  Multiport Switch1/1 -> yd_d/1  "yd_d"
  Trajetóra em 8/2(yd_d) -> Multiport Switch1/5  "yd_d"
  "Trajetóra em \"L\" Curva 180° suave RAMPA"/2(yd_d) -> Multiport Switch1/4  "yd_d"
  "Trajetóra em \"L\" Curva 180° suave RAMPA"/1(xd_d) -> Multiport Switch/4  "xd_d"
  Trajetóra em 8/1(xd_d) -> Multiport Switch/5

== system modelo_real/Trajetória Desejada/Velocidade da trajetória/Circulo ==
  Gain : Gain  Gain=w
  Gain1 : Gain  Gain=v
  Gain2 : Gain  Gain=w
  Gain3 : Gain  Gain=v
  Gain4 : Gain  Gain=-1
  Ramp18 : simulink/Sources/Ramp  slope=1  start=t_i  InitialOutput=0
  Ramp19 : simulink/Sources/Ramp  slope=-1  start=t_i  InitialOutput=0
  Trigonometric Function : Trigonometry
  Trigonometric Function1 : Trigonometry  Operator=cos
  xd_d : Outport
  yd_d : Outport  Port=2
  wires:
  Gain4/1 -> Gain1/1
  Ramp18/1 -> Gain/1
  Gain/1 -> Trigonometric Function/1
  Trigonometric Function1/1 -> Gain3/1
  Gain2/1 -> Trigonometric Function1/1
  Ramp19/1 -> Gain2/1
  Gain1/1 -> xd_d/1
  Gain3/1 -> yd_d/1
  Trigonometric Function/1 -> Gain4/1

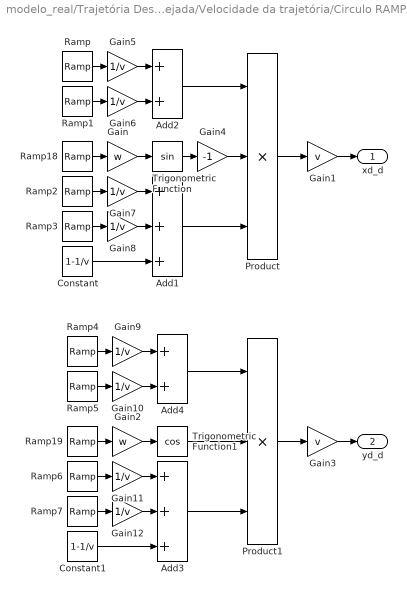
== system modelo_real/Trajetória Desejada/Velocidade da trajetória/Circulo RAMPA ==
  Add1 : Sum  Inputs=3
  Add2 : Sum  Inputs=2
  Add3 : Sum  Inputs=3
  Add4 : Sum  Inputs=2
  Constant : Constant  Value=1-1/v
  Constant1 : Constant  Value=1-1/v
  Gain : Gain  Gain=w
  Gain1 : Gain  Gain=v
  Gain{5..12} (8 alike) : Gain  Gain=1/v
  Gain2 : Gain  Gain=w
  Gain3 : Gain  Gain=v
  Gain4 : Gain  Gain=-1
  Product : Product  Inputs=3
  Product1 : Product  Inputs=3
  Ramp : simulink/Sources/Ramp  slope=a  start=t_i  InitialOutput=0
  Ramp1 : simulink/Sources/Ramp  slope=-a  start=t_1  InitialOutput=0
  Ramp18 : simulink/Sources/Ramp  slope=1  start=t_i  InitialOutput=0
  Ramp19 : simulink/Sources/Ramp  slope=1  start=t_i  InitialOutput=0
  Ramp2 : simulink/Sources/Ramp  slope=-a  start=t_2  InitialOutput=1
  Ramp3 : simulink/Sources/Ramp  slope=a  start=t_f  InitialOutput=0
  Ramp4 : simulink/Sources/Ramp  slope=a  start=t_i  InitialOutput=0
  Ramp5 : simulink/Sources/Ramp  slope=-a  start=t_1  InitialOutput=0
  Ramp6 : simulink/Sources/Ramp  slope=-a  start=t_2  InitialOutput=1
  Ramp7 : simulink/Sources/Ramp  slope=a  start=t_f  InitialOutput=0
  Trigonometric Function : Trigonometry
  Trigonometric Function1 : Trigonometry  Operator=cos
  xd_d : Outport
  yd_d : Outport  Port=2
  wires:
  Product/1 -> Gain1/1
  Ramp18/1 -> Gain/1
  Gain/1 -> Trigonometric Function/1
  Gain2/1 -> Trigonometric Function1/1
  Ramp19/1 -> Gain2/1
  Gain1/1 -> xd_d/1
  Gain3/1 -> yd_d/1
  Trigonometric Function/1 -> Gain4/1
  Ramp/1 -> Gain5/1
  Ramp1/1 -> Gain6/1
  Gain5/1 -> Add2/1
  Gain6/1 -> Add2/2
  Add2/1 -> Product/1
  Gain4/1 -> Product/2
  Product1/1 -> Gain3/1
  Trigonometric Function1/1 -> Product1/2
  Ramp2/1 -> Gain7/1
  Gain7/1 -> Add1/1
  Ramp3/1 -> Gain8/1
  Gain8/1 -> Add1/2
  Add1/1 -> Product/3
  Constant/1 -> Add1/3
  Ramp6/1 -> Gain11/1
  Add3/1 -> Product1/3
  Constant1/1 -> Add3/3
  Gain12/1 -> Add3/2
  Gain9/1 -> Add4/1
  Add4/1 -> Product1/1
  Gain11/1 -> Add3/1
  Ramp4/1 -> Gain9/1
  Ramp7/1 -> Gain12/1
  Gain10/1 -> Add4/2
  Ramp5/1 -> Gain10/1

== system modelo_real/Trajetória Desejada/Velocidade da trajetória/Linha Reta RAMPA ==
  Add1 : Sum
  Add2 : Sum  Inputs=++++++
  Constant : Constant  Value=0
  Gain1 : Gain  Gain=v
  Ramp : simulink/Sources/Ramp  slope=a  start=t_i  InitialOutput=0
  Ramp1 : simulink/Sources/Ramp  slope=-a  start=t_i_1  InitialOutput=0
  Ramp2 : simulink/Sources/Ramp  slope=-a  start=t_i_2  InitialOutput=0
  Step1 : Step  Time=t_i_1  After=-v  SampleTime=0
  Step18 : Step  Time=t_i_1  SampleTime=0
  Step19 : Step  Time=t_i_2  After=-1  SampleTime=0
  Step2 : Step  Time=t_i_2  After=v  SampleTime=0
  xd_d : Outport
  yd_d : Outport  Port=2
  wires:
  Add1/1 -> Gain1/1
  Step18/1 -> Add1/1
  Step19/1 -> Add1/2
  Add2/1 -> xd_d/1
  Ramp/1 -> Add2/1
  Ramp1/1 -> Add2/2
  Step1/1 -> Add2/3
  Gain1/1 -> Add2/4
  Ramp2/1 -> Add2/5
  Step2/1 -> Add2/6
  Constant/1 -> yd_d/1

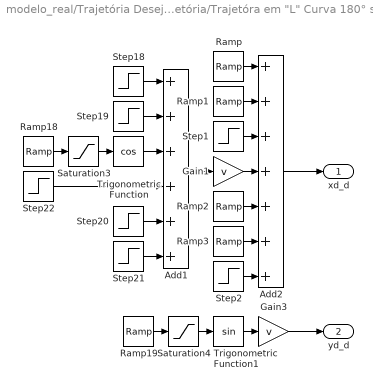
== system modelo_real/Trajetória Desejada/Velocidade da trajetória/Trajetóra em "L" Curva 180° suave RAMPA ==
  Add1 : Sum  Inputs=++++++
  Add2 : Sum  Inputs=+++++++
  Gain1 : Gain  Gain=v
  Gain3 : Gain  Gain=v
  Ramp : simulink/Sources/Ramp  slope=a  start=t_i  InitialOutput=0
  Ramp1 : simulink/Sources/Ramp  slope=-a  start=t_i_1  InitialOutput=0
  Ramp18 : simulink/Sources/Ramp  slope=pi/dur_c  start=t_i_c  InitialOutput=0
  Ramp19 : simulink/Sources/Ramp  slope=pi/dur_c  start=t_i_c  InitialOutput=0
  Ramp2 : simulink/Sources/Ramp  slope=a  start=t_i_3  InitialOutput=0
  Ramp3 : simulink/Sources/Ramp  slope=-a  start=t_f  InitialOutput=0
  Saturation3 : Saturate  UpperLimit=pi  LowerLimit=0
  Saturation4 : Saturate  UpperLimit=pi  LowerLimit=0
  Step1 : Step  Time=t_i_1  After=-v  SampleTime=0
  Step18 : Step  Time=t_i_1  SampleTime=0
  Step19 : Step  Time=t_i_c  After=-1  SampleTime=0
  Step2 : Step  Time=t_i_3  After=-v  SampleTime=0
  Step20 : Step  Time=t_i_3  SampleTime=0
  Step21 : Step  Time=t_f  After=-1  SampleTime=0
  Step22 : Step  Time=t_i_c  Before=-1  After=0  SampleTime=0
  Trigonometric Function : Trigonometry  Operator=cos
  Trigonometric Function1 : Trigonometry
  xd_d : Outport
  yd_d : Outport  Port=2
  wires:
  Add1/1 -> Gain1/1
  Ramp18/1 -> Saturation3/1
  Saturation3/1 -> Trigonometric Function/1
  Saturation4/1 -> Trigonometric Function1/1
  Ramp19/1 -> Saturation4/1
  Step18/1 -> Add1/1
  Step19/1 -> Add1/2
  Trigonometric Function/1 -> Add1/3
  Step22/1 -> Add1/4
  Add2/1 -> xd_d/1
  Ramp/1 -> Add2/1
  Ramp1/1 -> Add2/2
  Step1/1 -> Add2/3
  Gain1/1 -> Add2/4
  Gain3/1 -> yd_d/1
  Ramp2/1 -> Add2/5
  Ramp3/1 -> Add2/6
  Step20/1 -> Add1/5
  Step21/1 -> Add1/6
  Step2/1 -> Add2/7
  Trigonometric Function1/1 -> Gain3/1

== system modelo_real/Trajetória Desejada/Velocidade da trajetória/Trajetóra em "L" Curva 90° suave  ==
  Add7 : Sum  Inputs=++++
  Add8 : Sum  Inputs=++++
  Gain1 : Gain  Gain=v
  Gain3 : Gain  Gain=v
  Ramp18 : simulink/Sources/Ramp  slope=(pi/2)/time_c  start=t_i_c  InitialOutput=0
  Ramp19 : simulink/Sources/Ramp  slope=(pi/2)/time_c  start=t_i_c  InitialOutput=0
  Saturation3 : Saturate  UpperLimit=pi/2  LowerLimit=0
  Saturation4 : Saturate  UpperLimit=pi/2  LowerLimit=0
  Step18 : Step  Time=t_i  SampleTime=0
  Step19 : Step  Time=t_i_c  After=-1  SampleTime=0
  Step20 : Step  Time=t_i_2  SampleTime=0
  Step21 : Step  Time=t_f  After=-1  SampleTime=0
  Step22 : Step  Time=t_i_c  Before=-1  After=0  SampleTime=0
  Step23 : Step  Time=t_i_2  After=-1  SampleTime=0
  Trigonometric Function : Trigonometry  Operator=cos
  Trigonometric Function1 : Trigonometry
  xd_d : Outport
  yd_d : Outport  Port=2
  wires:
  Add7/1 -> Gain1/1
  Ramp18/1 -> Saturation3/1
  Step21/1 -> Add8/4
  Saturation3/1 -> Trigonometric Function/1
  Add8/1 -> Gain3/1
  Step20/1 -> Add8/3
  Trigonometric Function1/1 -> Add8/1
  Saturation4/1 -> Trigonometric Function1/1
  Ramp19/1 -> Saturation4/1
  Step23/1 -> Add8/2
  Gain1/1 -> xd_d/1
  Gain3/1 -> yd_d/1
  Step22/1 -> Add7/4
  Trigonometric Function/1 -> Add7/3
  Step19/1 -> Add7/2
  Step18/1 -> Add7/1

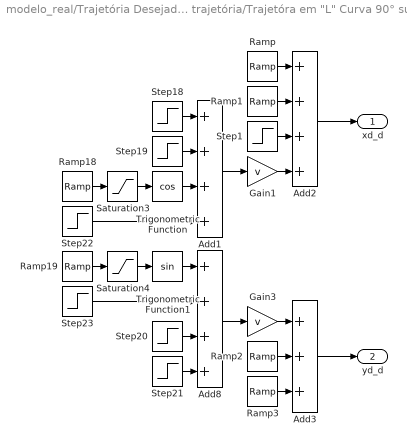
== system modelo_real/Trajetória Desejada/Velocidade da trajetória/Trajetóra em "L" Curva 90° suave RAMPA ==
  Add1 : Sum  Inputs=++++
  Add2 : Sum  Inputs=++++
  Add3 : Sum  Inputs=+++
  Add8 : Sum  Inputs=++++
  Gain1 : Gain  Gain=v
  Gain3 : Gain  Gain=v
  Ramp : simulink/Sources/Ramp  slope=a  start=t_i  InitialOutput=0
  Ramp1 : simulink/Sources/Ramp  slope=-a  start=t_i_1  InitialOutput=0
  Ramp18 : simulink/Sources/Ramp  slope=(pi/2)/dur_c  start=t_i_c  InitialOutput=0
  Ramp19 : simulink/Sources/Ramp  slope=(pi/2)/dur_c  start=t_i_c  InitialOutput=0
  Ramp2 : simulink/Sources/Ramp  slope=-a  start=t_i_3  InitialOutput=0
  Ramp3 : simulink/Sources/Ramp  slope=a  start=t_f  InitialOutput=0
  Saturation3 : Saturate  UpperLimit=pi/2  LowerLimit=0
  Saturation4 : Saturate  UpperLimit=pi/2  LowerLimit=0
  Step1 : Step  Time=t_i_1  After=-v  SampleTime=0
  Step18 : Step  Time=t_i_1  SampleTime=0
  Step19 : Step  Time=t_i_c  After=-1  SampleTime=0
  Step20 : Step  Time=t_i_2  SampleTime=0
  Step21 : Step  Time=t_f  After=-1  SampleTime=0
  Step22 : Step  Time=t_i_c  Before=-1  After=0  SampleTime=0
  Step23 : Step  Time=t_i_2  After=-1  SampleTime=0
  Trigonometric Function : Trigonometry  Operator=cos
  Trigonometric Function1 : Trigonometry
  xd_d : Outport
  yd_d : Outport  Port=2
  wires:
  Add1/1 -> Gain1/1
  Ramp18/1 -> Saturation3/1
  Step21/1 -> Add8/4
  Saturation3/1 -> Trigonometric Function/1
  Add8/1 -> Gain3/1
  Step20/1 -> Add8/3
  Trigonometric Function1/1 -> Add8/1
  Saturation4/1 -> Trigonometric Function1/1
  Ramp19/1 -> Saturation4/1
  Step23/1 -> Add8/2
  Step18/1 -> Add1/1
  Step19/1 -> Add1/2
  Trigonometric Function/1 -> Add1/3
  Step22/1 -> Add1/4
  Add2/1 -> xd_d/1
  Ramp/1 -> Add2/1
  Ramp1/1 -> Add2/2
  Step1/1 -> Add2/3
  Gain1/1 -> Add2/4
  Gain3/1 -> Add3/1
  Add3/1 -> yd_d/1
  Ramp2/1 -> Add3/2
  Ramp3/1 -> Add3/3

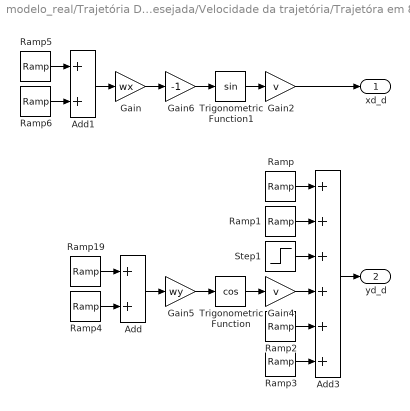
== system modelo_real/Trajetória Desejada/Velocidade da trajetória/Trajetóra em 8 ==
  Add : Sum
  Add1 : Sum
  Add3 : Sum  Inputs=++++++
  Gain : Gain  Gain=wx
  Gain2 : Gain  Gain=v
  Gain4 : Gain  Gain=v
  Gain5 : Gain  Gain=wy
  Gain6 : Gain  Gain=-1
  Ramp : simulink/Sources/Ramp  slope=a  start=t_i  InitialOutput=0
  Ramp1 : simulink/Sources/Ramp  slope=-a  start=t_i_1  InitialOutput=0
  Ramp19 : simulink/Sources/Ramp  slope=1  start=t_i_1  InitialOutput=0
  Ramp2 : simulink/Sources/Ramp  slope=-a  start=t_i_2  InitialOutput=0
  Ramp3 : simulink/Sources/Ramp  slope=a  start=t_f  InitialOutput=0
  Ramp4 : simulink/Sources/Ramp  slope=-1  start=t_i_2  InitialOutput=0
  Ramp5 : simulink/Sources/Ramp  slope=1  start=t_i_1  InitialOutput=0
  Ramp6 : simulink/Sources/Ramp  slope=-1  start=t_i_2  InitialOutput=0
  Step1 : Step  Time=t_i  After=-v  SampleTime=0
  Trigonometric Function : Trigonometry  Operator=cos
  Trigonometric Function1 : Trigonometry
  xd_d : Outport
  yd_d : Outport  Port=2
  wires:
  Add1/1 -> Gain/1
  Trigonometric Function/1 -> Gain4/1
  Trigonometric Function1/1 -> Gain2/1
  Add3/1 -> yd_d/1
  Gain/1 -> Gain6/1
  Gain5/1 -> Trigonometric Function/1
  Gain6/1 -> Trigonometric Function1/1
  Gain4/1 -> Add3/4
  Ramp2/1 -> Add3/5
  Ramp3/1 -> Add3/6
  Ramp1/1 -> Add3/2
  Ramp/1 -> Add3/1
  Step1/1 -> Add3/3
  Ramp19/1 -> Add/1
  Add/1 -> Gain5/1
  Ramp4/1 -> Add/2
  Ramp6/1 -> Add1/2
  Ramp5/1 -> Add1/1
  Gain2/1 -> xd_d/1

== matlab function modelo_real/Modelo Real/Obtenção dos estados/Cinemática diferencial ==
  data: cte input; thetaD input; x0_3 input; xo_d output; thetaD_d input; x0_5 input; thetaE input; x0_4 input; thetaE_d input; yo_d output; x3 output; x4 output; x5 output; x6 output; x0_6 input
function [xo_d, yo_d, x3, x4, x5, x6] = fcn(cte, thetaD, x0_3, thetaD_d, x0_5, thetaE, x0_4, thetaE_d, x0_6)

r_d = cte(1,1);
r_e = cte(1,2);
c_d = cte(1,3);
c_e = cte(1,4);

x3   = thetaD   + x0_3;
x4   = thetaE   + x0_4;
x5   = thetaD_d + x0_5;
x6   = thetaE_d + x0_6;

phi  = c_d*x3-c_e*x4;

xo_d = (r_d/2)*cos(phi)*x5 + (r_e/2)*cos(phi)*x6;
yo_d = (r_d/2)*sin(phi)*x5 + (r_e/2)*sin(phi)*x6;

== matlab function modelo_real/Modelo Real/Filtro D/Média ==
  data: u input; y output
function y = fcn(u)
y = mean(u);

== matlab function modelo_real/Modelo Real/Filtro E/Média ==
  data: u input; y output
function y = fcn(u)
y = mean(u);
